simulink model "model_sim_CHB5_36_new_temp"  (R2020a)
settings: Solver=FixedStepAuto  StartTime=0.0  StopTime=5  RelTol=1e-3
InitFcn:
  | sysinit
values from neighbouring files (symbols this model uses):
  C = 0.03    [sysinit.m]
  C_f = 0.625e-6    (= 6.25e-07)    [sysinit.m]
  f = 50    [sysinit.m]
  f_switch = 500    [sysinit.m]
  L = 0.004    [sysinit.m]
  L_f = 3e-6    (= 3e-06)    [sysinit.m]
  R = 1.2    [sysinit.m]
  R_f = 1.5    [sysinit.m]
  Rth_h = 7.5e-3    (= 0.0075)    [Device_Parameter.m]
  Rth_h_tau = 0.5    [Device_Parameter.m]
  st = 5e-7    (= 5e-07)    [sysinit.m]
  temp_init = 40    [sysinit.m]
  Ts = 1e-6    (= 1e-06)    [sysinit.m]
  Ts2 = 0.5E-3    (= 0.0005)    [sysinit.m]
  Udc = 2500    [sysinit.m]
undefined symbols (not defined in the file or in its folder): DIODE_204520, DIODE_344520, DIODE_D1031SH, DIODE_D1331SH, IGCT_364520_36, IGCT_364521_36, IGCT_654522_6, magnitude, Ts1
libraries: powerlib x278, powerlib_meascontrol x84, simulink x9
(part 2 of 5)

== system model_sim_CHB5_36_new_temp/MAIN TOPOLOGY level-5/IGCT4 ==
  PWM : Inport
  Current Measurement1 : powerlib/Measurements/Current Measurement  PhasorSimulation=off  OutputType=Complex  PSBequivalent=0
  Demux : Demux
  Diode{1..3,6,8} (5 alike) : powerlib/Power Electronics/Diode  Ron=rto  Lon=0  Vf=vto  IC=0  UseSnubber=off  Rs=500  Cs=250e-9  Measurements=on
  IGBT{,1..3} (4 alike) : powerlib/Power Electronics/IGBT  Ron=rt  Lon=0  Vf=vt  Tf=1e-6  Tt=2e-6  IC=0  Rs=1e5  Cs=inf  Measurements=on
  Series RLC Branch1 : powerlib/Elements/Series RLC Branch  LConnTagsString=__new0  RConnTagsString=__new0  BranchType=RL  Resistance=1e-5  Inductance=3.0E-6  SetiL0=off  InitialCurrent=0  Capacitance=1e-6  Setx0=off  InitialVoltage=0  Measurements=None
  Series RLC Branch10 : powerlib/Elements/Series RLC Branch  LConnTagsString=__new0  RConnTagsString=__new0  BranchType=L  Resistance=1  Inductance=0.4e-6  SetiL0=off  InitialCurrent=0  Capacitance=1e-6  Setx0=off  InitialVoltage=0  Measurements=None
  Series RLC Branch12 : powerlib/Elements/Series RLC Branch  LConnTagsString=__new0  RConnTagsString=__new0  BranchType=RL  Resistance=1e-5  Inductance=1E-9  SetiL0=off  InitialCurrent=0  Capacitance=1e-6  Setx0=off  InitialVoltage=0  Measurements=None
  Series RLC Branch14 : powerlib/Elements/Series RLC Branch  LConnTagsString=__new0  RConnTagsString=__new0  BranchType=L  Resistance=1  Inductance=1E-7  SetiL0=off  InitialCurrent=0  Capacitance=1e-6  Setx0=off  InitialVoltage=0  Measurements=None
  Series RLC Branch2 : powerlib/Elements/Series RLC Branch  LConnTagsString=__new0  RConnTagsString=__new0  BranchType=RC  Resistance=1e-5  Inductance=20e-6  SetiL0=off  InitialCurrent=0  Capacitance=17e-6  Setx0=off  InitialVoltage=0  Measurements=None
  Series RLC Branch3 : powerlib/Elements/Series RLC Branch  LConnTagsString=__new0  RConnTagsString=__new0  BranchType=RL  Resistance=1e-5  Inductance=1E-9  SetiL0=off  InitialCurrent=0  Capacitance=1e-6  Setx0=off  InitialVoltage=0  Measurements=None
  Series RLC Branch5 : powerlib/Elements/Series RLC Branch  LConnTagsString=__new0  RConnTagsString=__new0  BranchType=L  Resistance=1  Inductance=1E-7  SetiL0=off  InitialCurrent=0  Capacitance=1e-6  Setx0=off  InitialVoltage=0  Measurements=None
  Series RLC Branch7 : powerlib/Elements/Series RLC Branch  LConnTagsString=__new0  RConnTagsString=__new0  BranchType=RL  Resistance=0.6  Inductance=1e-6  SetiL0=off  InitialCurrent=0  Capacitance=1e-6  Setx0=off  InitialVoltage=0  Measurements=None
  Series RLC Branch9 : powerlib/Elements/Series RLC Branch  LConnTagsString=__new0  RConnTagsString=__new0  BranchType=L  Resistance=1  Inductance=0.4e-6  SetiL0=off  InitialCurrent=0  Capacitance=1e-6  Setx0=off  InitialVoltage=0  Measurements=None
  Terminator{,1..9} (10 alike) : Terminator
  Udc+ : PMIOPort  Side=Left
  udc- : PMIOPort  Port=2  Side=Left
  p1 : PMIOPort  Port=3  Side=Right
  p2 : PMIOPort  Port=4  Side=Right
  wires:
  Diode3/1 -> Terminator9/1
  IGBT3/1 -> Terminator5/1
  [n1] -> IGBT3/1
  IGBT1/1 -> Terminator4/1
  IGBT2/1 -> Terminator3/1
  IGBT/1 -> Terminator2/1
  [n2] -> IGBT1/1
  [p1] -> IGBT2/1
  Current Measurement1/1 -> Terminator/1
  Diode2/1 -> Terminator8/1
  [p2] -> IGBT/1
  Diode8/1 -> Terminator7/1
  Diode1/1 -> Terminator6/1
  Diode6/1 -> Terminator1/1
  Demux/3 -> [n2]
  PWM/1 -> Demux/1
  Demux/1 -> [p2]
  Demux/2 -> [p1]
  Demux/4 -> [n1]
  connections:
  Series RLC Branch10/LConn1 -- udc-/RConn1
  Series RLC Branch9/LConn1 -- Udc+/RConn1
  Diode6/RConn1 -- Series RLC Branch7/RConn1 -- Series RLC Branch2/LConn1
  Current Measurement1/LConn1 -- Series RLC Branch1/RConn1 -- Series RLC Branch3/LConn1 -- Series RLC Branch12/LConn1
  Diode3/LConn1 -- IGBT3/RConn1 -- Series RLC Branch14/RConn1
  Series RLC Branch3/RConn1 -- IGBT/LConn1 -- Diode8/RConn1
  Diode1/LConn1 -- Series RLC Branch5/RConn1 -- IGBT1/RConn1
  Current Measurement1/RConn1 -- Diode6/LConn1
  Diode2/RConn1 -- Series RLC Branch12/RConn1 -- IGBT2/LConn1
  p1/RConn1 -- Diode2/LConn1 -- Diode3/RConn1 -- IGBT3/LConn1 -- IGBT2/RConn1
  Series RLC Branch5/LConn1 -- Series RLC Branch14/LConn1 -- Series RLC Branch10/RConn1 -- Series RLC Branch2/RConn1
  Series RLC Branch1/LConn1 -- Series RLC Branch7/LConn1 -- Series RLC Branch9/RConn1
  p2/RConn1 -- IGBT1/LConn1 -- Diode1/RConn1 -- Diode8/LConn1 -- IGBT/RConn1

== system model_sim_CHB5_36_new_temp/MAIN TOPOLOGY level-5/IGCT5 ==
  PWM : Inport
  Current Measurement1 : powerlib/Measurements/Current Measurement  PhasorSimulation=off  OutputType=Complex  PSBequivalent=0
  Demux : Demux
  Diode{1..3,6,8} (5 alike) : powerlib/Power Electronics/Diode  Ron=rto  Lon=0  Vf=vto  IC=0  UseSnubber=off  Rs=500  Cs=250e-9  Measurements=on
  IGBT{,1..3} (4 alike) : powerlib/Power Electronics/IGBT  Ron=rt  Lon=0  Vf=vt  Tf=1e-6  Tt=2e-6  IC=0  Rs=1e5  Cs=inf  Measurements=on
  Series RLC Branch1 : powerlib/Elements/Series RLC Branch  LConnTagsString=__new0  RConnTagsString=__new0  BranchType=RL  Resistance=1e-5  Inductance=3.0E-6  SetiL0=off  InitialCurrent=0  Capacitance=1e-6  Setx0=off  InitialVoltage=0  Measurements=None
  Series RLC Branch10 : powerlib/Elements/Series RLC Branch  LConnTagsString=__new0  RConnTagsString=__new0  BranchType=L  Resistance=1  Inductance=0.4e-6  SetiL0=off  InitialCurrent=0  Capacitance=1e-6  Setx0=off  InitialVoltage=0  Measurements=None
  Series RLC Branch12 : powerlib/Elements/Series RLC Branch  LConnTagsString=__new0  RConnTagsString=__new0  BranchType=RL  Resistance=1e-5  Inductance=1E-9  SetiL0=off  InitialCurrent=0  Capacitance=1e-6  Setx0=off  InitialVoltage=0  Measurements=None
  Series RLC Branch14 : powerlib/Elements/Series RLC Branch  LConnTagsString=__new0  RConnTagsString=__new0  BranchType=L  Resistance=1  Inductance=1E-7  SetiL0=off  InitialCurrent=0  Capacitance=1e-6  Setx0=off  InitialVoltage=0  Measurements=None
  Series RLC Branch2 : powerlib/Elements/Series RLC Branch  LConnTagsString=__new0  RConnTagsString=__new0  BranchType=RC  Resistance=1e-5  Inductance=20e-6  SetiL0=off  InitialCurrent=0  Capacitance=17e-6  Setx0=off  InitialVoltage=0  Measurements=None
  Series RLC Branch3 : powerlib/Elements/Series RLC Branch  LConnTagsString=__new0  RConnTagsString=__new0  BranchType=RL  Resistance=1e-5  Inductance=1E-9  SetiL0=off  InitialCurrent=0  Capacitance=1e-6  Setx0=off  InitialVoltage=0  Measurements=None
  Series RLC Branch5 : powerlib/Elements/Series RLC Branch  LConnTagsString=__new0  RConnTagsString=__new0  BranchType=L  Resistance=1  Inductance=1E-7  SetiL0=off  InitialCurrent=0  Capacitance=1e-6  Setx0=off  InitialVoltage=0  Measurements=None
  Series RLC Branch7 : powerlib/Elements/Series RLC Branch  LConnTagsString=__new0  RConnTagsString=__new0  BranchType=RL  Resistance=0.6  Inductance=1e-6  SetiL0=off  InitialCurrent=0  Capacitance=1e-6  Setx0=off  InitialVoltage=0  Measurements=None
  Series RLC Branch9 : powerlib/Elements/Series RLC Branch  LConnTagsString=__new0  RConnTagsString=__new0  BranchType=L  Resistance=1  Inductance=0.4e-6  SetiL0=off  InitialCurrent=0  Capacitance=1e-6  Setx0=off  InitialVoltage=0  Measurements=None
  Terminator{,1..9} (10 alike) : Terminator
  Udc+ : PMIOPort  Side=Left
  udc- : PMIOPort  Port=2  Side=Left
  p1 : PMIOPort  Port=3  Side=Right
  p2 : PMIOPort  Port=4  Side=Right
  wires:
  Diode3/1 -> Terminator9/1
  IGBT3/1 -> Terminator5/1
  [n1] -> IGBT3/1
  IGBT1/1 -> Terminator4/1
  IGBT2/1 -> Terminator3/1
  IGBT/1 -> Terminator2/1
  [n2] -> IGBT1/1
  [p1] -> IGBT2/1
  Current Measurement1/1 -> Terminator/1
  Diode2/1 -> Terminator8/1
  [p2] -> IGBT/1
  Diode8/1 -> Terminator7/1
  Diode1/1 -> Terminator6/1
  Diode6/1 -> Terminator1/1
  Demux/3 -> [n2]
  PWM/1 -> Demux/1
  Demux/1 -> [p2]
  Demux/2 -> [p1]
  Demux/4 -> [n1]
  connections:
  Series RLC Branch10/LConn1 -- udc-/RConn1
  Series RLC Branch9/LConn1 -- Udc+/RConn1
  Diode6/RConn1 -- Series RLC Branch7/RConn1 -- Series RLC Branch2/LConn1
  Current Measurement1/LConn1 -- Series RLC Branch1/RConn1 -- Series RLC Branch3/LConn1 -- Series RLC Branch12/LConn1
  Diode3/LConn1 -- IGBT3/RConn1 -- Series RLC Branch14/RConn1
  Series RLC Branch3/RConn1 -- IGBT/LConn1 -- Diode8/RConn1
  Diode1/LConn1 -- Series RLC Branch5/RConn1 -- IGBT1/RConn1
  Current Measurement1/RConn1 -- Diode6/LConn1
  Diode2/RConn1 -- Series RLC Branch12/RConn1 -- IGBT2/LConn1
  p1/RConn1 -- Diode2/LConn1 -- Diode3/RConn1 -- IGBT3/LConn1 -- IGBT2/RConn1
  Series RLC Branch5/LConn1 -- Series RLC Branch14/LConn1 -- Series RLC Branch10/RConn1 -- Series RLC Branch2/RConn1
  Series RLC Branch1/LConn1 -- Series RLC Branch7/LConn1 -- Series RLC Branch9/RConn1
  p2/RConn1 -- IGBT1/LConn1 -- Diode1/RConn1 -- Diode8/LConn1 -- IGBT/RConn1

== system model_sim_CHB5_36_new_temp/MAIN TOPOLOGY level-5/IGCT6 ==
  PWM : Inport
  Current Measurement1 : powerlib/Measurements/Current Measurement  PhasorSimulation=off  OutputType=Complex  PSBequivalent=0
  Demux : Demux
  Diode{1..3,6,8} (5 alike) : powerlib/Power Electronics/Diode  Ron=rto  Lon=0  Vf=vto  IC=0  UseSnubber=off  Rs=500  Cs=250e-9  Measurements=on
  IGBT{,1..3} (4 alike) : powerlib/Power Electronics/IGBT  Ron=rt  Lon=0  Vf=vt  Tf=1e-6  Tt=2e-6  IC=0  Rs=1e5  Cs=inf  Measurements=on
  Series RLC Branch1 : powerlib/Elements/Series RLC Branch  LConnTagsString=__new0  RConnTagsString=__new0  BranchType=RL  Resistance=1e-5  Inductance=3.0E-6  SetiL0=off  InitialCurrent=0  Capacitance=1e-6  Setx0=off  InitialVoltage=0  Measurements=None
  Series RLC Branch10 : powerlib/Elements/Series RLC Branch  LConnTagsString=__new0  RConnTagsString=__new0  BranchType=L  Resistance=1  Inductance=0.4e-6  SetiL0=off  InitialCurrent=0  Capacitance=1e-6  Setx0=off  InitialVoltage=0  Measurements=None
  Series RLC Branch12 : powerlib/Elements/Series RLC Branch  LConnTagsString=__new0  RConnTagsString=__new0  BranchType=RL  Resistance=1e-5  Inductance=1E-9  SetiL0=off  InitialCurrent=0  Capacitance=1e-6  Setx0=off  InitialVoltage=0  Measurements=None
  Series RLC Branch14 : powerlib/Elements/Series RLC Branch  LConnTagsString=__new0  RConnTagsString=__new0  BranchType=L  Resistance=1  Inductance=1E-7  SetiL0=off  InitialCurrent=0  Capacitance=1e-6  Setx0=off  InitialVoltage=0  Measurements=None
  Series RLC Branch2 : powerlib/Elements/Series RLC Branch  LConnTagsString=__new0  RConnTagsString=__new0  BranchType=RC  Resistance=1e-5  Inductance=20e-6  SetiL0=off  InitialCurrent=0  Capacitance=17e-6  Setx0=off  InitialVoltage=0  Measurements=None
  Series RLC Branch3 : powerlib/Elements/Series RLC Branch  LConnTagsString=__new0  RConnTagsString=__new0  BranchType=RL  Resistance=1e-5  Inductance=1E-9  SetiL0=off  InitialCurrent=0  Capacitance=1e-6  Setx0=off  InitialVoltage=0  Measurements=None
  Series RLC Branch5 : powerlib/Elements/Series RLC Branch  LConnTagsString=__new0  RConnTagsString=__new0  BranchType=L  Resistance=1  Inductance=1E-7  SetiL0=off  InitialCurrent=0  Capacitance=1e-6  Setx0=off  InitialVoltage=0  Measurements=None
  Series RLC Branch7 : powerlib/Elements/Series RLC Branch  LConnTagsString=__new0  RConnTagsString=__new0  BranchType=RL  Resistance=0.6  Inductance=1e-6  SetiL0=off  InitialCurrent=0  Capacitance=1e-6  Setx0=off  InitialVoltage=0  Measurements=None
  Series RLC Branch9 : powerlib/Elements/Series RLC Branch  LConnTagsString=__new0  RConnTagsString=__new0  BranchType=L  Resistance=1  Inductance=0.4e-6  SetiL0=off  InitialCurrent=0  Capacitance=1e-6  Setx0=off  InitialVoltage=0  Measurements=None
  Terminator{,1..9} (10 alike) : Terminator
  Udc+ : PMIOPort  Side=Left
  udc- : PMIOPort  Port=2  Side=Left
  p1 : PMIOPort  Port=3  Side=Right
  p2 : PMIOPort  Port=4  Side=Right
  wires:
  Demux/4 -> [n1]
  Demux/2 -> [p1]
  Demux/1 -> [p2]
  PWM/1 -> Demux/1
  Demux/3 -> [n2]
  Diode6/1 -> Terminator1/1
  Diode1/1 -> Terminator6/1
  Diode8/1 -> Terminator7/1
  [p2] -> IGBT/1
  Diode2/1 -> Terminator8/1
  Current Measurement1/1 -> Terminator/1
  [p1] -> IGBT2/1
  [n2] -> IGBT1/1
  IGBT/1 -> Terminator2/1
  IGBT2/1 -> Terminator3/1
  IGBT1/1 -> Terminator4/1
  [n1] -> IGBT3/1
  IGBT3/1 -> Terminator5/1
  Diode3/1 -> Terminator9/1
  connections:
  IGBT/RConn1 -- Diode8/LConn1 -- Diode1/RConn1 -- IGBT1/LConn1 -- p2/RConn1
  Series RLC Branch9/RConn1 -- Series RLC Branch7/LConn1 -- Series RLC Branch1/LConn1
  Series RLC Branch2/RConn1 -- Series RLC Branch10/RConn1 -- Series RLC Branch14/LConn1 -- Series RLC Branch5/LConn1
  IGBT2/RConn1 -- IGBT3/LConn1 -- Diode3/RConn1 -- Diode2/LConn1 -- p1/RConn1
  IGBT2/LConn1 -- Series RLC Branch12/RConn1 -- Diode2/RConn1
  Current Measurement1/RConn1 -- Diode6/LConn1
  IGBT1/RConn1 -- Series RLC Branch5/RConn1 -- Diode1/LConn1
  Diode8/RConn1 -- IGBT/LConn1 -- Series RLC Branch3/RConn1
  Series RLC Branch14/RConn1 -- IGBT3/RConn1 -- Diode3/LConn1
  Series RLC Branch12/LConn1 -- Series RLC Branch3/LConn1 -- Series RLC Branch1/RConn1 -- Current Measurement1/LConn1
  Series RLC Branch2/LConn1 -- Series RLC Branch7/RConn1 -- Diode6/RConn1
  Series RLC Branch9/LConn1 -- Udc+/RConn1
  Series RLC Branch10/LConn1 -- udc-/RConn1

== system model_sim_CHB5_36_new_temp/MAIN TOPOLOGY level-5/Subsystem2 ==
  Zigzag Phase-Shifting Transformer : powerlib/Elements/Zigzag Phase-Shifting Transformer  SecondaryConnection=Delta D1(-30 deg.)  SetSaturation=off  SetInitialFlux=off  Measurements=None  UNITS=pu  NominalPower=[ p 50]  PrimaryVoltage=vp  SecondaryVoltage="[ vs  +5]"  Winding1=windingpri  Winding2=windingpri  Winding3=windingsec  RmLm=mag  Rm=500  Saturation=[ 0,0 ; 0.0024,1.2 ; 1.0,1.52 ]  InitialFluxes=[0,0,0]  BreakLoop=off  DiscreteSolver=Trapezoidal iterative  DataType=off
  Zigzag Phase-Shifting Transformer1 : powerlib/Elements/Zigzag Phase-Shifting Transformer  SecondaryConnection=Delta D1(-30 deg.)  SetSaturation=off  SetInitialFlux=off  Measurements=None  UNITS=pu  NominalPower=[ p 50]  PrimaryVoltage=vp  SecondaryVoltage="[ vs  +15]"  Winding1=windingpri  Winding2=windingpri  Winding3=windingsec  RmLm=mag  Rm=500  Saturation=[ 0,0 ; 0.0024,1.2 ; 1.0,1.52 ]  InitialFluxes=[0,0,0]  BreakLoop=off  DiscreteSolver=Trapezoidal iterative  DataType=off
  Zigzag Phase-Shifting Transformer2 : powerlib/Elements/Zigzag Phase-Shifting Transformer  SecondaryConnection=Delta D1(-30 deg.)  SetSaturation=off  SetInitialFlux=off  Measurements=None  UNITS=pu  NominalPower=[ p 50]  PrimaryVoltage=vp  SecondaryVoltage="[ vs  +25]"  Winding1=windingpri  Winding2=windingpri  Winding3=windingsec  RmLm=mag  Rm=500  Saturation=[ 0,0 ; 0.0024,1.2 ; 1.0,1.52 ]  InitialFluxes=[0,0,0]  BreakLoop=off  DiscreteSolver=Trapezoidal iterative  DataType=off
  Zigzag Phase-Shifting Transformer3 : powerlib/Elements/Zigzag Phase-Shifting Transformer  SecondaryConnection=Delta D1(-30 deg.)  SetSaturation=off  SetInitialFlux=off  Measurements=None  UNITS=pu  NominalPower=[ p 50]  PrimaryVoltage=vp  SecondaryVoltage="[ vs  -25]"  Winding1=windingpri  Winding2=windingpri  Winding3=windingsec  RmLm=mag  Rm=500  Saturation=[ 0,0 ; 0.0024,1.2 ; 1.0,1.52 ]  InitialFluxes=[0,0,0]  BreakLoop=off  DiscreteSolver=Trapezoidal iterative  DataType=off
  Zigzag Phase-Shifting Transformer4 : powerlib/Elements/Zigzag Phase-Shifting Transformer  SecondaryConnection=Delta D1(-30 deg.)  SetSaturation=off  SetInitialFlux=off  Measurements=None  UNITS=pu  NominalPower=[ p 50]  PrimaryVoltage=vp  SecondaryVoltage="[ vs  -5]"  Winding1=windingpri  Winding2=windingpri  Winding3=windingsec  RmLm=mag  Rm=500  Saturation=[ 0,0 ; 0.0024,1.2 ; 1.0,1.52 ]  InitialFluxes=[0,0,0]  BreakLoop=off  DiscreteSolver=Trapezoidal iterative  DataType=off
  Zigzag Phase-Shifting Transformer5 : powerlib/Elements/Zigzag Phase-Shifting Transformer  SecondaryConnection=Delta D1(-30 deg.)  SetSaturation=off  SetInitialFlux=off  Measurements=None  UNITS=pu  NominalPower=[ p 50]  PrimaryVoltage=vp  SecondaryVoltage="[ vs  -15]"  Winding1=windingpri  Winding2=windingpri  Winding3=windingsec  RmLm=mag  Rm=500  Saturation=[ 0,0 ; 0.0024,1.2 ; 1.0,1.52 ]  InitialFluxes=[0,0,0]  BreakLoop=off  DiscreteSolver=Trapezoidal iterative  DataType=off
  output Ground1 : powerlib/Elements/Ground  LConnTagsString=a  RConnTagsString=__newr0
  A : PMIOPort  Side=Left
  a+5 : PMIOPort  Port=2  Side=Right
  B : PMIOPort  Port=3  Side=Left
  C : PMIOPort  Port=4  Side=Left
  b+5 : PMIOPort  Port=5  Side=Right
  c+5 : PMIOPort  Port=6  Side=Right
  a-25 : PMIOPort  Port=7  Side=Right
  b-25 : PMIOPort  Port=8  Side=Right
  c-25 : PMIOPort  Port=9  Side=Right
  a+15 : PMIOPort  Port=10  Side=Right
  b+15 : PMIOPort  Port=11  Side=Right
  c+15 : PMIOPort  Port=12  Side=Right
  a-15 : PMIOPort  Port=13  Side=Right
  b-15 : PMIOPort  Port=14  Side=Right
  c-15 : PMIOPort  Port=15  Side=Right
  a25 : PMIOPort  Port=16  Side=Right
  b25 : PMIOPort  Port=17  Side=Right
  c25 : PMIOPort  Port=18  Side=Right
  a-5 : PMIOPort  Port=19  Side=Right
  b-5 : PMIOPort  Port=20  Side=Right
  c-5 : PMIOPort  Port=21  Side=Right
  connections:
  Zigzag Phase-Shifting Transformer4/LConn4 -- Zigzag Phase-Shifting Transformer4/LConn5 -- output Ground1/LConn1 -- Zigzag Phase-Shifting Transformer4/LConn6
  b+5/RConn1 -- Zigzag Phase-Shifting Transformer/RConn2
  a+5/RConn1 -- Zigzag Phase-Shifting Transformer/RConn1
  c+5/RConn1 -- Zigzag Phase-Shifting Transformer/RConn3
  c-25/RConn1 -- Zigzag Phase-Shifting Transformer3/RConn3
  b-25/RConn1 -- Zigzag Phase-Shifting Transformer3/RConn2
  a-25/RConn1 -- Zigzag Phase-Shifting Transformer3/RConn1
  c+15/RConn1 -- Zigzag Phase-Shifting Transformer1/RConn3
  b+15/RConn1 -- Zigzag Phase-Shifting Transformer1/RConn2
  a+15/RConn1 -- Zigzag Phase-Shifting Transformer1/RConn1
  c-15/RConn1 -- Zigzag Phase-Shifting Transformer5/RConn3
  b-15/RConn1 -- Zigzag Phase-Shifting Transformer5/RConn2
  a-15/RConn1 -- Zigzag Phase-Shifting Transformer5/RConn1
  c25/RConn1 -- Zigzag Phase-Shifting Transformer2/RConn3
  b25/RConn1 -- Zigzag Phase-Shifting Transformer2/RConn2
  a25/RConn1 -- Zigzag Phase-Shifting Transformer2/RConn1
  c-5/RConn1 -- Zigzag Phase-Shifting Transformer4/RConn3
  b-5/RConn1 -- Zigzag Phase-Shifting Transformer4/RConn2
  a-5/RConn1 -- Zigzag Phase-Shifting Transformer4/RConn1
  Zigzag Phase-Shifting Transformer2/LConn6 -- Zigzag Phase-Shifting Transformer4/LConn3
  Zigzag Phase-Shifting Transformer3/LConn6 -- Zigzag Phase-Shifting Transformer1/LConn3
  Zigzag Phase-Shifting Transformer1/LConn6 -- Zigzag Phase-Shifting Transformer5/LConn3
  Zigzag Phase-Shifting Transformer5/LConn6 -- Zigzag Phase-Shifting Transformer2/LConn3
  Zigzag Phase-Shifting Transformer/LConn2 -- B/RConn1
  Zigzag Phase-Shifting Transformer/LConn4 -- Zigzag Phase-Shifting Transformer3/LConn1
  Zigzag Phase-Shifting Transformer/LConn5 -- Zigzag Phase-Shifting Transformer3/LConn2
  Zigzag Phase-Shifting Transformer/LConn6 -- Zigzag Phase-Shifting Transformer3/LConn3
  Zigzag Phase-Shifting Transformer3/LConn4 -- Zigzag Phase-Shifting Transformer1/LConn1
  Zigzag Phase-Shifting Transformer3/LConn5 -- Zigzag Phase-Shifting Transformer1/LConn2
  Zigzag Phase-Shifting Transformer1/LConn4 -- Zigzag Phase-Shifting Transformer5/LConn1
  Zigzag Phase-Shifting Transformer1/LConn5 -- Zigzag Phase-Shifting Transformer5/LConn2
  Zigzag Phase-Shifting Transformer5/LConn4 -- Zigzag Phase-Shifting Transformer2/LConn1
  Zigzag Phase-Shifting Transformer5/LConn5 -- Zigzag Phase-Shifting Transformer2/LConn2
  Zigzag Phase-Shifting Transformer2/LConn4 -- Zigzag Phase-Shifting Transformer4/LConn1
  Zigzag Phase-Shifting Transformer4/LConn2 -- Zigzag Phase-Shifting Transformer2/LConn5
  C/RConn1 -- Zigzag Phase-Shifting Transformer/LConn3
  A/RConn1 -- Zigzag Phase-Shifting Transformer/LConn1

== system model_sim_CHB5_36_new_temp/MAIN TOPOLOGY level-5/VOLTAGE_MEASURE ==
  Voltage Measurement{1..6} (6 alike) : powerlib/Measurements/Voltage Measurement  PhasorSimulation=off  OutputType=Complex  PSBequivalent=0
  N : PMIOPort  Side=Left
  A : PMIOPort  Port=2  Side=Left
  B : PMIOPort  Port=3  Side=Right
  C : PMIOPort  Port=4  Side=Right
  tag scope: VloadABline=global, VloadAphase=global, VloadBCline=global, VloadBphase=global, VloadCAline=global, VloadCphase=global
  wires:
  Voltage Measurement2/1 -> [VloadAphase]
  Voltage Measurement4/1 -> [VloadBphase]
  Voltage Measurement5/1 -> [VloadCAline]
  Voltage Measurement3/1 -> [VloadBCline]
  Voltage Measurement1/1 -> [VloadABline]
  Voltage Measurement6/1 -> [VloadCphase]
  connections:
  Voltage Measurement2/LConn2 -- Voltage Measurement6/LConn2 -- Voltage Measurement4/LConn2 -- N/RConn1
  Voltage Measurement6/LConn1 -- Voltage Measurement5/LConn1 -- Voltage Measurement3/LConn2 -- C/RConn1
  Voltage Measurement3/LConn1 -- Voltage Measurement1/LConn2 -- B/RConn1 -- Voltage Measurement4/LConn1
  Voltage Measurement5/LConn2 -- Voltage Measurement1/LConn1 -- Voltage Measurement2/LConn1 -- A/RConn1

== system model_sim_CHB5_36_new_temp/Subsystem/IGCT1 ==
  PWM : Inport
  Current Measurement1 : powerlib/Measurements/Current Measurement  PhasorSimulation=off  OutputType=Complex  PSBequivalent=0
  Demux : Demux
  Diode{1..3,6,8} (5 alike) : powerlib/Power Electronics/Diode  Ron=DIODE.rF  Lon=0  Vf=DIODE.VF0  IC=0  UseSnubber=off  Rs=500  Cs=250e-9  Measurements=on
  IGBT{,1..3} (4 alike) : powerlib/Power Electronics/IGBT  Ron=IGCT.rT  Lon=0  Vf=IGCT.VT0  Tf=1e-6  Tt=2e-6  IC=0  Rs=1e5  Cs=inf  Measurements=on
  Series RLC Branch1 : powerlib/Elements/Series RLC Branch  LConnTagsString=__new0  RConnTagsString=__new0  BranchType=RL  Resistance=1e-5  Inductance=3.0E-6  SetiL0=off  InitialCurrent=0  Capacitance=1e-6  Setx0=off  InitialVoltage=0  Measurements=None
  Series RLC Branch10 : powerlib/Elements/Series RLC Branch  LConnTagsString=__new0  RConnTagsString=__new0  BranchType=L  Resistance=1  Inductance=0.4e-6  SetiL0=off  InitialCurrent=0  Capacitance=1e-6  Setx0=off  InitialVoltage=0  Measurements=None
  Series RLC Branch12 : powerlib/Elements/Series RLC Branch  LConnTagsString=__new0  RConnTagsString=__new0  BranchType=RL  Resistance=1e-5  Inductance=1E-9  SetiL0=off  InitialCurrent=0  Capacitance=1e-6  Setx0=off  InitialVoltage=0  Measurements=None
  Series RLC Branch14 : powerlib/Elements/Series RLC Branch  LConnTagsString=__new0  RConnTagsString=__new0  BranchType=L  Resistance=1  Inductance=1E-7  SetiL0=off  InitialCurrent=0  Capacitance=1e-6  Setx0=off  InitialVoltage=0  Measurements=None
  Series RLC Branch2 : powerlib/Elements/Series RLC Branch  LConnTagsString=__new0  RConnTagsString=__new0  BranchType=RC  Resistance=1e-5  Inductance=20e-6  SetiL0=off  InitialCurrent=0  Capacitance=17e-6  Setx0=off  InitialVoltage=0  Measurements=None
  Series RLC Branch3 : powerlib/Elements/Series RLC Branch  LConnTagsString=__new0  RConnTagsString=__new0  BranchType=RL  Resistance=1e-5  Inductance=1E-9  SetiL0=off  InitialCurrent=0  Capacitance=1e-6  Setx0=off  InitialVoltage=0  Measurements=None
  Series RLC Branch5 : powerlib/Elements/Series RLC Branch  LConnTagsString=__new0  RConnTagsString=__new0  BranchType=L  Resistance=1  Inductance=1E-7  SetiL0=off  InitialCurrent=0  Capacitance=1e-6  Setx0=off  InitialVoltage=0  Measurements=None
  Series RLC Branch7 : powerlib/Elements/Series RLC Branch  LConnTagsString=__new0  RConnTagsString=__new0  BranchType=RL  Resistance=0.6  Inductance=1e-6  SetiL0=off  InitialCurrent=0  Capacitance=1e-6  Setx0=off  InitialVoltage=0  Measurements=None
  Series RLC Branch9 : powerlib/Elements/Series RLC Branch  LConnTagsString=__new0  RConnTagsString=__new0  BranchType=L  Resistance=1  Inductance=0.4e-6  SetiL0=off  InitialCurrent=0  Capacitance=1e-6  Setx0=off  InitialVoltage=0  Measurements=None
  Terminator{,1..9} (10 alike) : Terminator
  Udc+ : PMIOPort  Side=Left
  udc- : PMIOPort  Port=2  Side=Left
  p1 : PMIOPort  Port=3  Side=Right
  p2 : PMIOPort  Port=4  Side=Right
  wires:
  Diode3/1 -> Terminator9/1
  IGBT3/1 -> Terminator5/1
  [n1] -> IGBT3/1
  IGBT1/1 -> Terminator4/1
  IGBT2/1 -> Terminator3/1
  IGBT/1 -> Terminator2/1
  [n2] -> IGBT1/1
  [p1] -> IGBT2/1
  Current Measurement1/1 -> Terminator/1
  Diode2/1 -> Terminator8/1
  [p2] -> IGBT/1
  Diode8/1 -> Terminator7/1
  Diode1/1 -> Terminator6/1
  Diode6/1 -> Terminator1/1
  Demux/3 -> [n2]
  PWM/1 -> Demux/1
  Demux/1 -> [p2]
  Demux/2 -> [p1]
  Demux/4 -> [n1]
  connections:
  Series RLC Branch10/LConn1 -- udc-/RConn1
  Series RLC Branch9/LConn1 -- Udc+/RConn1
  Diode6/RConn1 -- Series RLC Branch7/RConn1 -- Series RLC Branch2/LConn1
  Current Measurement1/LConn1 -- Series RLC Branch1/RConn1 -- Series RLC Branch3/LConn1 -- Series RLC Branch12/LConn1
  Series RLC Branch14/RConn1 -- Diode3/LConn1 -- IGBT3/RConn1
  Series RLC Branch3/RConn1 -- IGBT/LConn1 -- Diode8/RConn1
  Series RLC Branch5/RConn1 -- Diode1/LConn1 -- IGBT1/RConn1
  Current Measurement1/RConn1 -- Diode6/LConn1
  Series RLC Branch12/RConn1 -- IGBT2/LConn1 -- Diode2/RConn1
  p1/RConn1 -- Diode3/RConn1 -- IGBT3/LConn1 -- IGBT2/RConn1 -- Diode2/LConn1
  Series RLC Branch5/LConn1 -- Series RLC Branch14/LConn1 -- Series RLC Branch10/RConn1 -- Series RLC Branch2/RConn1
  Series RLC Branch1/LConn1 -- Series RLC Branch7/LConn1 -- Series RLC Branch9/RConn1
  p2/RConn1 -- Diode1/RConn1 -- IGBT1/LConn1 -- Diode8/LConn1 -- IGBT/RConn1

== system model_sim_CHB5_36_new_temp/Subsystem/IGCT2 ==
  PWM : Inport
  Current Measurement1 : powerlib/Measurements/Current Measurement  PhasorSimulation=off  OutputType=Complex  PSBequivalent=0
  Demux : Demux
  Diode{1..3,6,8} (5 alike) : powerlib/Power Electronics/Diode  Ron=DIODE.rF  Lon=0  Vf=DIODE.VF0  IC=0  UseSnubber=off  Rs=500  Cs=250e-9  Measurements=on
  IGBT{,1..3} (4 alike) : powerlib/Power Electronics/IGBT  Ron=IGCT.rT  Lon=0  Vf=IGCT.VT0  Tf=1e-6  Tt=2e-6  IC=0  Rs=1e5  Cs=inf  Measurements=on
  Series RLC Branch1 : powerlib/Elements/Series RLC Branch  LConnTagsString=__new0  RConnTagsString=__new0  BranchType=RL  Resistance=1e-5  Inductance=3.0E-6  SetiL0=off  InitialCurrent=0  Capacitance=1e-6  Setx0=off  InitialVoltage=0  Measurements=None
  Series RLC Branch10 : powerlib/Elements/Series RLC Branch  LConnTagsString=__new0  RConnTagsString=__new0  BranchType=L  Resistance=1  Inductance=0.4e-6  SetiL0=off  InitialCurrent=0  Capacitance=1e-6  Setx0=off  InitialVoltage=0  Measurements=None
  Series RLC Branch12 : powerlib/Elements/Series RLC Branch  LConnTagsString=__new0  RConnTagsString=__new0  BranchType=RL  Resistance=1e-5  Inductance=1E-9  SetiL0=off  InitialCurrent=0  Capacitance=1e-6  Setx0=off  InitialVoltage=0  Measurements=None
  Series RLC Branch14 : powerlib/Elements/Series RLC Branch  LConnTagsString=__new0  RConnTagsString=__new0  BranchType=L  Resistance=1  Inductance=1E-7  SetiL0=off  InitialCurrent=0  Capacitance=1e-6  Setx0=off  InitialVoltage=0  Measurements=None
  Series RLC Branch2 : powerlib/Elements/Series RLC Branch  LConnTagsString=__new0  RConnTagsString=__new0  BranchType=RC  Resistance=1e-5  Inductance=20e-6  SetiL0=off  InitialCurrent=0  Capacitance=17e-6  Setx0=off  InitialVoltage=0  Measurements=None
  Series RLC Branch3 : powerlib/Elements/Series RLC Branch  LConnTagsString=__new0  RConnTagsString=__new0  BranchType=RL  Resistance=1e-5  Inductance=1E-9  SetiL0=off  InitialCurrent=0  Capacitance=1e-6  Setx0=off  InitialVoltage=0  Measurements=None
  Series RLC Branch5 : powerlib/Elements/Series RLC Branch  LConnTagsString=__new0  RConnTagsString=__new0  BranchType=L  Resistance=1  Inductance=1E-7  SetiL0=off  InitialCurrent=0  Capacitance=1e-6  Setx0=off  InitialVoltage=0  Measurements=None
  Series RLC Branch7 : powerlib/Elements/Series RLC Branch  LConnTagsString=__new0  RConnTagsString=__new0  BranchType=RL  Resistance=0.6  Inductance=1e-6  SetiL0=off  InitialCurrent=0  Capacitance=1e-6  Setx0=off  InitialVoltage=0  Measurements=None
  Series RLC Branch9 : powerlib/Elements/Series RLC Branch  LConnTagsString=__new0  RConnTagsString=__new0  BranchType=L  Resistance=1  Inductance=0.4e-6  SetiL0=off  InitialCurrent=0  Capacitance=1e-6  Setx0=off  InitialVoltage=0  Measurements=None
  Terminator{,1..9} (10 alike) : Terminator
  Udc+ : PMIOPort  Side=Left
  udc- : PMIOPort  Port=2  Side=Left
  p1 : PMIOPort  Port=3  Side=Right
  p2 : PMIOPort  Port=4  Side=Right
  wires:
  Demux/4 -> [n1]
  Demux/2 -> [p1]
  Demux/1 -> [p2]
  PWM/1 -> Demux/1
  Demux/3 -> [n2]
  Diode6/1 -> Terminator1/1
  Diode1/1 -> Terminator6/1
  Diode8/1 -> Terminator7/1
  [p2] -> IGBT/1
  Diode2/1 -> Terminator8/1
  Current Measurement1/1 -> Terminator/1
  [p1] -> IGBT2/1
  [n2] -> IGBT1/1
  IGBT/1 -> Terminator2/1
  IGBT2/1 -> Terminator3/1
  IGBT1/1 -> Terminator4/1
  [n1] -> IGBT3/1
  IGBT3/1 -> Terminator5/1
  Diode3/1 -> Terminator9/1
  connections:
  Diode1/RConn1 -- IGBT/RConn1 -- Diode8/LConn1 -- p2/RConn1 -- IGBT1/LConn1
  Series RLC Branch9/RConn1 -- Series RLC Branch7/LConn1 -- Series RLC Branch1/LConn1
  Series RLC Branch2/RConn1 -- Series RLC Branch10/RConn1 -- Series RLC Branch14/LConn1 -- Series RLC Branch5/LConn1
  Diode3/RConn1 -- IGBT2/RConn1 -- IGBT3/LConn1 -- p1/RConn1 -- Diode2/LConn1
  IGBT2/LConn1 -- Series RLC Branch12/RConn1 -- Diode2/RConn1
  Current Measurement1/RConn1 -- Diode6/LConn1
  Diode1/LConn1 -- Series RLC Branch5/RConn1 -- IGBT1/RConn1
  Diode8/RConn1 -- IGBT/LConn1 -- Series RLC Branch3/RConn1
  Diode3/LConn1 -- Series RLC Branch14/RConn1 -- IGBT3/RConn1
  Series RLC Branch12/LConn1 -- Series RLC Branch3/LConn1 -- Series RLC Branch1/RConn1 -- Current Measurement1/LConn1
  Series RLC Branch2/LConn1 -- Series RLC Branch7/RConn1 -- Diode6/RConn1
  Series RLC Branch9/LConn1 -- Udc+/RConn1
  Series RLC Branch10/LConn1 -- udc-/RConn1

== system model_sim_CHB5_36_new_temp/Subsystem/IGCT3 ==
  PWM : Inport
  Current Measurement1 : powerlib/Measurements/Current Measurement  PhasorSimulation=off  OutputType=Complex  PSBequivalent=0
  Demux : Demux
  Diode{1..3,6,8} (5 alike) : powerlib/Power Electronics/Diode  Ron=DIODE.rF  Lon=0  Vf=DIODE.VF0  IC=0  UseSnubber=off  Rs=500  Cs=250e-9  Measurements=on
  IGBT{,1..3} (4 alike) : powerlib/Power Electronics/IGBT  Ron=IGCT.rT  Lon=0  Vf=IGCT.VT0  Tf=1e-6  Tt=2e-6  IC=0  Rs=1e5  Cs=inf  Measurements=on
  Series RLC Branch1 : powerlib/Elements/Series RLC Branch  LConnTagsString=__new0  RConnTagsString=__new0  BranchType=RL  Resistance=1e-5  Inductance=3.0E-6  SetiL0=off  InitialCurrent=0  Capacitance=1e-6  Setx0=off  InitialVoltage=0  Measurements=None
  Series RLC Branch10 : powerlib/Elements/Series RLC Branch  LConnTagsString=__new0  RConnTagsString=__new0  BranchType=L  Resistance=1  Inductance=0.4e-6  SetiL0=off  InitialCurrent=0  Capacitance=1e-6  Setx0=off  InitialVoltage=0  Measurements=None
  Series RLC Branch12 : powerlib/Elements/Series RLC Branch  LConnTagsString=__new0  RConnTagsString=__new0  BranchType=RL  Resistance=1e-5  Inductance=1E-9  SetiL0=off  InitialCurrent=0  Capacitance=1e-6  Setx0=off  InitialVoltage=0  Measurements=None
  Series RLC Branch14 : powerlib/Elements/Series RLC Branch  LConnTagsString=__new0  RConnTagsString=__new0  BranchType=L  Resistance=1  Inductance=1E-7  SetiL0=off  InitialCurrent=0  Capacitance=1e-6  Setx0=off  InitialVoltage=0  Measurements=None
  Series RLC Branch2 : powerlib/Elements/Series RLC Branch  LConnTagsString=__new0  RConnTagsString=__new0  BranchType=RC  Resistance=1e-5  Inductance=20e-6  SetiL0=off  InitialCurrent=0  Capacitance=17e-6  Setx0=off  InitialVoltage=0  Measurements=None
  Series RLC Branch3 : powerlib/Elements/Series RLC Branch  LConnTagsString=__new0  RConnTagsString=__new0  BranchType=RL  Resistance=1e-5  Inductance=1E-9  SetiL0=off  InitialCurrent=0  Capacitance=1e-6  Setx0=off  InitialVoltage=0  Measurements=None
  Series RLC Branch5 : powerlib/Elements/Series RLC Branch  LConnTagsString=__new0  RConnTagsString=__new0  BranchType=L  Resistance=1  Inductance=1E-7  SetiL0=off  InitialCurrent=0  Capacitance=1e-6  Setx0=off  InitialVoltage=0  Measurements=None
  Series RLC Branch7 : powerlib/Elements/Series RLC Branch  LConnTagsString=__new0  RConnTagsString=__new0  BranchType=RL  Resistance=0.6  Inductance=1e-6  SetiL0=off  InitialCurrent=0  Capacitance=1e-6  Setx0=off  InitialVoltage=0  Measurements=None
  Series RLC Branch9 : powerlib/Elements/Series RLC Branch  LConnTagsString=__new0  RConnTagsString=__new0  BranchType=L  Resistance=1  Inductance=0.4e-6  SetiL0=off  InitialCurrent=0  Capacitance=1e-6  Setx0=off  InitialVoltage=0  Measurements=None
  Terminator{,1..9} (10 alike) : Terminator
  Udc+ : PMIOPort  Side=Left
  udc- : PMIOPort  Port=2  Side=Left
  p1 : PMIOPort  Port=3  Side=Right
  p2 : PMIOPort  Port=4  Side=Right
  wires:
  Diode3/1 -> Terminator9/1
  IGBT3/1 -> Terminator5/1
  [n1] -> IGBT3/1
  IGBT1/1 -> Terminator4/1
  IGBT2/1 -> Terminator3/1
  IGBT/1 -> Terminator2/1
  [n2] -> IGBT1/1
  [p1] -> IGBT2/1
  Current Measurement1/1 -> Terminator/1
  Diode2/1 -> Terminator8/1
  [p2] -> IGBT/1
  Diode8/1 -> Terminator7/1
  Diode1/1 -> Terminator6/1
  Diode6/1 -> Terminator1/1
  Demux/3 -> [n2]
  PWM/1 -> Demux/1
  Demux/1 -> [p2]
  Demux/2 -> [p1]
  Demux/4 -> [n1]
  connections:
  Series RLC Branch10/LConn1 -- udc-/RConn1
  Series RLC Branch9/LConn1 -- Udc+/RConn1
  Diode6/RConn1 -- Series RLC Branch7/RConn1 -- Series RLC Branch2/LConn1
  Current Measurement1/LConn1 -- Series RLC Branch1/RConn1 -- Series RLC Branch3/LConn1 -- Series RLC Branch12/LConn1
  IGBT3/RConn1 -- Series RLC Branch14/RConn1 -- Diode3/LConn1
  Series RLC Branch3/RConn1 -- IGBT/LConn1 -- Diode8/RConn1
  IGBT1/RConn1 -- Series RLC Branch5/RConn1 -- Diode1/LConn1
  Current Measurement1/RConn1 -- Diode6/LConn1
  Diode2/RConn1 -- Series RLC Branch12/RConn1 -- IGBT2/LConn1
  Diode2/LConn1 -- p1/RConn1 -- IGBT3/LConn1 -- IGBT2/RConn1 -- Diode3/RConn1
  Series RLC Branch5/LConn1 -- Series RLC Branch14/LConn1 -- Series RLC Branch10/RConn1 -- Series RLC Branch2/RConn1
  Series RLC Branch1/LConn1 -- Series RLC Branch7/LConn1 -- Series RLC Branch9/RConn1
  IGBT1/LConn1 -- p2/RConn1 -- Diode8/LConn1 -- IGBT/RConn1 -- Diode1/RConn1

== system model_sim_CHB5_36_new_temp/Subsystem/IGCT4 ==
  PWM : Inport
  Current Measurement1 : powerlib/Measurements/Current Measurement  PhasorSimulation=off  OutputType=Complex  PSBequivalent=0
  Demux : Demux
  Diode{1..3,6,8} (5 alike) : powerlib/Power Electronics/Diode  Ron=DIODE.rF  Lon=0  Vf=DIODE.VF0  IC=0  UseSnubber=off  Rs=500  Cs=250e-9  Measurements=on
  IGBT{,1..3} (4 alike) : powerlib/Power Electronics/IGBT  Ron=IGCT.rT  Lon=0  Vf=IGCT.VT0  Tf=1e-6  Tt=2e-6  IC=0  Rs=1e5  Cs=inf  Measurements=on
  Series RLC Branch1 : powerlib/Elements/Series RLC Branch  LConnTagsString=__new0  RConnTagsString=__new0  BranchType=RL  Resistance=1e-5  Inductance=3.0E-6  SetiL0=off  InitialCurrent=0  Capacitance=1e-6  Setx0=off  InitialVoltage=0  Measurements=None
  Series RLC Branch10 : powerlib/Elements/Series RLC Branch  LConnTagsString=__new0  RConnTagsString=__new0  BranchType=L  Resistance=1  Inductance=0.4e-6  SetiL0=off  InitialCurrent=0  Capacitance=1e-6  Setx0=off  InitialVoltage=0  Measurements=None
  Series RLC Branch12 : powerlib/Elements/Series RLC Branch  LConnTagsString=__new0  RConnTagsString=__new0  BranchType=RL  Resistance=1e-5  Inductance=1E-9  SetiL0=off  InitialCurrent=0  Capacitance=1e-6  Setx0=off  InitialVoltage=0  Measurements=None
  Series RLC Branch14 : powerlib/Elements/Series RLC Branch  LConnTagsString=__new0  RConnTagsString=__new0  BranchType=L  Resistance=1  Inductance=1E-7  SetiL0=off  InitialCurrent=0  Capacitance=1e-6  Setx0=off  InitialVoltage=0  Measurements=None
  Series RLC Branch2 : powerlib/Elements/Series RLC Branch  LConnTagsString=__new0  RConnTagsString=__new0  BranchType=RC  Resistance=1e-5  Inductance=20e-6  SetiL0=off  InitialCurrent=0  Capacitance=17e-6  Setx0=off  InitialVoltage=0  Measurements=None
  Series RLC Branch3 : powerlib/Elements/Series RLC Branch  LConnTagsString=__new0  RConnTagsString=__new0  BranchType=RL  Resistance=1e-5  Inductance=1E-9  SetiL0=off  InitialCurrent=0  Capacitance=1e-6  Setx0=off  InitialVoltage=0  Measurements=None
  Series RLC Branch5 : powerlib/Elements/Series RLC Branch  LConnTagsString=__new0  RConnTagsString=__new0  BranchType=L  Resistance=1  Inductance=1E-7  SetiL0=off  InitialCurrent=0  Capacitance=1e-6  Setx0=off  InitialVoltage=0  Measurements=None
  Series RLC Branch7 : powerlib/Elements/Series RLC Branch  LConnTagsString=__new0  RConnTagsString=__new0  BranchType=RL  Resistance=0.6  Inductance=1e-6  SetiL0=off  InitialCurrent=0  Capacitance=1e-6  Setx0=off  InitialVoltage=0  Measurements=None
  Series RLC Branch9 : powerlib/Elements/Series RLC Branch  LConnTagsString=__new0  RConnTagsString=__new0  BranchType=L  Resistance=1  Inductance=0.4e-6  SetiL0=off  InitialCurrent=0  Capacitance=1e-6  Setx0=off  InitialVoltage=0  Measurements=None
  Terminator{,1..9} (10 alike) : Terminator
  Udc+ : PMIOPort  Side=Left
  udc- : PMIOPort  Port=2  Side=Left
  p1 : PMIOPort  Port=3  Side=Right
  p2 : PMIOPort  Port=4  Side=Right
  wires:
  Demux/4 -> [n1]
  Demux/2 -> [p1]
  Demux/1 -> [p2]
  PWM/1 -> Demux/1
  Demux/3 -> [n2]
  Diode6/1 -> Terminator1/1
  Diode1/1 -> Terminator6/1
  Diode8/1 -> Terminator7/1
  [p2] -> IGBT/1
  Diode2/1 -> Terminator8/1
  Current Measurement1/1 -> Terminator/1
  [p1] -> IGBT2/1
  [n2] -> IGBT1/1
  IGBT/1 -> Terminator2/1
  IGBT2/1 -> Terminator3/1
  IGBT1/1 -> Terminator4/1
  [n1] -> IGBT3/1
  IGBT3/1 -> Terminator5/1
  Diode3/1 -> Terminator9/1
  connections:
  Diode1/RConn1 -- IGBT/RConn1 -- Diode8/LConn1 -- p2/RConn1 -- IGBT1/LConn1
  Series RLC Branch9/RConn1 -- Series RLC Branch7/LConn1 -- Series RLC Branch1/LConn1
  Series RLC Branch2/RConn1 -- Series RLC Branch10/RConn1 -- Series RLC Branch14/LConn1 -- Series RLC Branch5/LConn1
  Diode3/RConn1 -- IGBT2/RConn1 -- IGBT3/LConn1 -- p1/RConn1 -- Diode2/LConn1
  IGBT2/LConn1 -- Series RLC Branch12/RConn1 -- Diode2/RConn1
  Current Measurement1/RConn1 -- Diode6/LConn1
  Diode1/LConn1 -- Series RLC Branch5/RConn1 -- IGBT1/RConn1
  Diode8/RConn1 -- IGBT/LConn1 -- Series RLC Branch3/RConn1
  Diode3/LConn1 -- Series RLC Branch14/RConn1 -- IGBT3/RConn1
  Series RLC Branch12/LConn1 -- Series RLC Branch3/LConn1 -- Series RLC Branch1/RConn1 -- Current Measurement1/LConn1
  Series RLC Branch2/LConn1 -- Series RLC Branch7/RConn1 -- Diode6/RConn1
  Series RLC Branch9/LConn1 -- Udc+/RConn1
  Series RLC Branch10/LConn1 -- udc-/RConn1

== system model_sim_CHB5_36_new_temp/Subsystem/IGCT5 ==
  PWM : Inport
  Current Measurement1 : powerlib/Measurements/Current Measurement  PhasorSimulation=off  OutputType=Complex  PSBequivalent=0
  Demux : Demux
  Diode{1..3,6,8} (5 alike) : powerlib/Power Electronics/Diode  Ron=DIODE.rF  Lon=0  Vf=DIODE.VF0  IC=0  UseSnubber=off  Rs=500  Cs=250e-9  Measurements=on
  IGBT{,1..3} (4 alike) : powerlib/Power Electronics/IGBT  Ron=IGCT.rT  Lon=0  Vf=IGCT.VT0  Tf=1e-6  Tt=2e-6  IC=0  Rs=1e5  Cs=inf  Measurements=on
  Series RLC Branch1 : powerlib/Elements/Series RLC Branch  LConnTagsString=__new0  RConnTagsString=__new0  BranchType=RL  Resistance=1e-5  Inductance=3.0E-6  SetiL0=off  InitialCurrent=0  Capacitance=1e-6  Setx0=off  InitialVoltage=0  Measurements=None
  Series RLC Branch10 : powerlib/Elements/Series RLC Branch  LConnTagsString=__new0  RConnTagsString=__new0  BranchType=L  Resistance=1  Inductance=0.4e-6  SetiL0=off  InitialCurrent=0  Capacitance=1e-6  Setx0=off  InitialVoltage=0  Measurements=None
  Series RLC Branch12 : powerlib/Elements/Series RLC Branch  LConnTagsString=__new0  RConnTagsString=__new0  BranchType=RL  Resistance=1e-5  Inductance=1E-9  SetiL0=off  InitialCurrent=0  Capacitance=1e-6  Setx0=off  InitialVoltage=0  Measurements=None
  Series RLC Branch14 : powerlib/Elements/Series RLC Branch  LConnTagsString=__new0  RConnTagsString=__new0  BranchType=L  Resistance=1  Inductance=1E-7  SetiL0=off  InitialCurrent=0  Capacitance=1e-6  Setx0=off  InitialVoltage=0  Measurements=None
  Series RLC Branch2 : powerlib/Elements/Series RLC Branch  LConnTagsString=__new0  RConnTagsString=__new0  BranchType=RC  Resistance=1e-5  Inductance=20e-6  SetiL0=off  InitialCurrent=0  Capacitance=17e-6  Setx0=off  InitialVoltage=0  Measurements=None
  Series RLC Branch3 : powerlib/Elements/Series RLC Branch  LConnTagsString=__new0  RConnTagsString=__new0  BranchType=RL  Resistance=1e-5  Inductance=1E-9  SetiL0=off  InitialCurrent=0  Capacitance=1e-6  Setx0=off  InitialVoltage=0  Measurements=None
  Series RLC Branch5 : powerlib/Elements/Series RLC Branch  LConnTagsString=__new0  RConnTagsString=__new0  BranchType=L  Resistance=1  Inductance=1E-7  SetiL0=off  InitialCurrent=0  Capacitance=1e-6  Setx0=off  InitialVoltage=0  Measurements=None
  Series RLC Branch7 : powerlib/Elements/Series RLC Branch  LConnTagsString=__new0  RConnTagsString=__new0  BranchType=RL  Resistance=0.6  Inductance=1e-6  SetiL0=off  InitialCurrent=0  Capacitance=1e-6  Setx0=off  InitialVoltage=0  Measurements=None
  Series RLC Branch9 : powerlib/Elements/Series RLC Branch  LConnTagsString=__new0  RConnTagsString=__new0  BranchType=L  Resistance=1  Inductance=0.4e-6  SetiL0=off  InitialCurrent=0  Capacitance=1e-6  Setx0=off  InitialVoltage=0  Measurements=None
  Terminator{,1..9} (10 alike) : Terminator
  Udc+ : PMIOPort  Side=Left
  udc- : PMIOPort  Port=2  Side=Left
  p1 : PMIOPort  Port=3  Side=Right
  p2 : PMIOPort  Port=4  Side=Right
  wires:
  Diode3/1 -> Terminator9/1
  IGBT3/1 -> Terminator5/1
  [n1] -> IGBT3/1
  IGBT1/1 -> Terminator4/1
  IGBT2/1 -> Terminator3/1
  IGBT/1 -> Terminator2/1
  [n2] -> IGBT1/1
  [p1] -> IGBT2/1
  Current Measurement1/1 -> Terminator/1
  Diode2/1 -> Terminator8/1
  [p2] -> IGBT/1
  Diode8/1 -> Terminator7/1
  Diode1/1 -> Terminator6/1
  Diode6/1 -> Terminator1/1
  Demux/3 -> [n2]
  PWM/1 -> Demux/1
  Demux/1 -> [p2]
  Demux/2 -> [p1]
  Demux/4 -> [n1]
  connections:
  Series RLC Branch10/LConn1 -- udc-/RConn1
  Series RLC Branch9/LConn1 -- Udc+/RConn1
  Diode6/RConn1 -- Series RLC Branch7/RConn1 -- Series RLC Branch2/LConn1
  Current Measurement1/LConn1 -- Series RLC Branch1/RConn1 -- Series RLC Branch3/LConn1 -- Series RLC Branch12/LConn1
  IGBT3/RConn1 -- Series RLC Branch14/RConn1 -- Diode3/LConn1
  Series RLC Branch3/RConn1 -- IGBT/LConn1 -- Diode8/RConn1
  IGBT1/RConn1 -- Series RLC Branch5/RConn1 -- Diode1/LConn1
  Current Measurement1/RConn1 -- Diode6/LConn1
  Diode2/RConn1 -- Series RLC Branch12/RConn1 -- IGBT2/LConn1
  Diode2/LConn1 -- p1/RConn1 -- IGBT3/LConn1 -- IGBT2/RConn1 -- Diode3/RConn1
  Series RLC Branch5/LConn1 -- Series RLC Branch14/LConn1 -- Series RLC Branch10/RConn1 -- Series RLC Branch2/RConn1
  Series RLC Branch1/LConn1 -- Series RLC Branch7/LConn1 -- Series RLC Branch9/RConn1
  IGBT1/LConn1 -- p2/RConn1 -- Diode8/LConn1 -- IGBT/RConn1 -- Diode1/RConn1

== system model_sim_CHB5_36_new_temp/Subsystem/IGCT6 ==
  PWM : Inport
  Current Measurement1 : powerlib/Measurements/Current Measurement  PhasorSimulation=off  OutputType=Complex  PSBequivalent=0
  Demux : Demux
  Diode{1..3,6,8} (5 alike) : powerlib/Power Electronics/Diode  Ron=DIODE.rF  Lon=0  Vf=DIODE.VF0  IC=0  UseSnubber=off  Rs=500  Cs=250e-9  Measurements=on
  IGBT{,1..3} (4 alike) : powerlib/Power Electronics/IGBT  Ron=IGCT.rT  Lon=0  Vf=IGCT.VT0  Tf=1e-6  Tt=2e-6  IC=0  Rs=1e5  Cs=inf  Measurements=on
  Series RLC Branch1 : powerlib/Elements/Series RLC Branch  LConnTagsString=__new0  RConnTagsString=__new0  BranchType=RL  Resistance=1e-5  Inductance=3.0E-6  SetiL0=off  InitialCurrent=0  Capacitance=1e-6  Setx0=off  InitialVoltage=0  Measurements=None
  Series RLC Branch10 : powerlib/Elements/Series RLC Branch  LConnTagsString=__new0  RConnTagsString=__new0  BranchType=L  Resistance=1  Inductance=0.4e-6  SetiL0=off  InitialCurrent=0  Capacitance=1e-6  Setx0=off  InitialVoltage=0  Measurements=None
  Series RLC Branch12 : powerlib/Elements/Series RLC Branch  LConnTagsString=__new0  RConnTagsString=__new0  BranchType=RL  Resistance=1e-5  Inductance=1E-9  SetiL0=off  InitialCurrent=0  Capacitance=1e-6  Setx0=off  InitialVoltage=0  Measurements=None
  Series RLC Branch14 : powerlib/Elements/Series RLC Branch  LConnTagsString=__new0  RConnTagsString=__new0  BranchType=L  Resistance=1  Inductance=1E-7  SetiL0=off  InitialCurrent=0  Capacitance=1e-6  Setx0=off  InitialVoltage=0  Measurements=None
  Series RLC Branch2 : powerlib/Elements/Series RLC Branch  LConnTagsString=__new0  RConnTagsString=__new0  BranchType=RC  Resistance=1e-5  Inductance=20e-6  SetiL0=off  InitialCurrent=0  Capacitance=17e-6  Setx0=off  InitialVoltage=0  Measurements=None
  Series RLC Branch3 : powerlib/Elements/Series RLC Branch  LConnTagsString=__new0  RConnTagsString=__new0  BranchType=RL  Resistance=1e-5  Inductance=1E-9  SetiL0=off  InitialCurrent=0  Capacitance=1e-6  Setx0=off  InitialVoltage=0  Measurements=None
  Series RLC Branch5 : powerlib/Elements/Series RLC Branch  LConnTagsString=__new0  RConnTagsString=__new0  BranchType=L  Resistance=1  Inductance=1E-7  SetiL0=off  InitialCurrent=0  Capacitance=1e-6  Setx0=off  InitialVoltage=0  Measurements=None
  Series RLC Branch7 : powerlib/Elements/Series RLC Branch  LConnTagsString=__new0  RConnTagsString=__new0  BranchType=RL  Resistance=0.6  Inductance=1e-6  SetiL0=off  InitialCurrent=0  Capacitance=1e-6  Setx0=off  InitialVoltage=0  Measurements=None
  Series RLC Branch9 : powerlib/Elements/Series RLC Branch  LConnTagsString=__new0  RConnTagsString=__new0  BranchType=L  Resistance=1  Inductance=0.4e-6  SetiL0=off  InitialCurrent=0  Capacitance=1e-6  Setx0=off  InitialVoltage=0  Measurements=None
  Terminator{,1..9} (10 alike) : Terminator
  Udc+ : PMIOPort  Side=Left
  udc- : PMIOPort  Port=2  Side=Left
  p1 : PMIOPort  Port=3  Side=Right
  p2 : PMIOPort  Port=4  Side=Right
  wires:
  Demux/4 -> [n1]
  Demux/2 -> [p1]
  Demux/1 -> [p2]
  PWM/1 -> Demux/1
  Demux/3 -> [n2]
  Diode6/1 -> Terminator1/1
  Diode1/1 -> Terminator6/1
  Diode8/1 -> Terminator7/1
  [p2] -> IGBT/1
  Diode2/1 -> Terminator8/1
  Current Measurement1/1 -> Terminator/1
  [p1] -> IGBT2/1
  [n2] -> IGBT1/1
  IGBT/1 -> Terminator2/1
  IGBT2/1 -> Terminator3/1
  IGBT1/1 -> Terminator4/1
  [n1] -> IGBT3/1
  IGBT3/1 -> Terminator5/1
  Diode3/1 -> Terminator9/1
  connections:
  Diode1/RConn1 -- IGBT/RConn1 -- Diode8/LConn1 -- p2/RConn1 -- IGBT1/LConn1
  Series RLC Branch9/RConn1 -- Series RLC Branch7/LConn1 -- Series RLC Branch1/LConn1
  Series RLC Branch2/RConn1 -- Series RLC Branch10/RConn1 -- Series RLC Branch14/LConn1 -- Series RLC Branch5/LConn1
  Diode3/RConn1 -- IGBT2/RConn1 -- IGBT3/LConn1 -- p1/RConn1 -- Diode2/LConn1
  IGBT2/LConn1 -- Series RLC Branch12/RConn1 -- Diode2/RConn1
  Current Measurement1/RConn1 -- Diode6/LConn1
  Diode1/LConn1 -- Series RLC Branch5/RConn1 -- IGBT1/RConn1
  Diode8/RConn1 -- IGBT/LConn1 -- Series RLC Branch3/RConn1
  Diode3/LConn1 -- Series RLC Branch14/RConn1 -- IGBT3/RConn1
  Series RLC Branch12/LConn1 -- Series RLC Branch3/LConn1 -- Series RLC Branch1/RConn1 -- Current Measurement1/LConn1
  Series RLC Branch2/LConn1 -- Series RLC Branch7/RConn1 -- Diode6/RConn1
  Series RLC Branch9/LConn1 -- Udc+/RConn1
  Series RLC Branch10/LConn1 -- udc-/RConn1

== system model_sim_CHB5_36_new_temp/Subsystem3/DIODE ==
  I : Inport
  PWM1 : Inport  Port=2
  PWM2 : Inport  Port=3
  PWM3 : Inport  Port=4
  PWM4 : Inport  Port=5
  DIODE_204520 : Subsystem  VariantControl=DIODE_TP ==1  mask{DIODE=DIODE_204520}
      mask DialogControl ParameterGroupVar Prompt: DEVICE
  DIODE_344520 : Subsystem  VariantControl=DIODE_TP ==2  mask{DIODE=DIODE_344520}
      mask DialogControl ParameterGroupVar Prompt: DEVICE
  DIODE_D1031SH : Subsystem  VariantControl=DIODE_TP ==3  mask{DIODE=DIODE_D1031SH}
      mask DialogControl ParameterGroupVar Prompt: DEVICE
  DIODE_D1331SH : Subsystem  VariantControl=DIODE_TP ==4  mask{DIODE=DIODE_D1331SH}
      mask DialogControl ParameterGroupVar Prompt: DEVICE
  D1_BUS : Outport
  D2_BUS : Outport  Port=2
  D1_LOSS_MEAN : Outport  Port=3
  D2_LOSS_MEAN : Outport  Port=4
  D1_TEMP : Outport  Port=5
  D2_TEMP : Outport  Port=6
  TEMLIM_BOOL : Outport  Port=7

== system model_sim_CHB5_36_new_temp/Subsystem3/IGCT ==
  I : Inport
  PWM1 : Inport  Port=2
  PWM2 : Inport  Port=3
  IGCT_364520_36 : Subsystem  VariantControl=IGCTTP == 1  mask{IGCT=IGCT_364520_36}
      mask DialogControl ParameterGroupVar Prompt: DEVICE
  IGCT_364521_36 : Subsystem  VariantControl=IGCTTP == 2  mask{IGCT=IGCT_364521_36}
      mask DialogControl ParameterGroupVar Prompt: DEVICE
  IGCT_654522_6 : Subsystem  VariantControl=IGCTTP == 3  mask{IGCT=IGCT_654522_6}
      mask DialogControl ParameterGroupVar Prompt: DEVICE
  T1_BUS : Outport
  T2_BUS : Outport  Port=2
  <T1_TEMP> : Outport  Port=3
  <T2_TEMP> : Outport  Port=4
  <T1_LOSS_MEAN> : Outport  Port=5
  <T2_LOSS_MEAN> : Outport  Port=6
  TEMLIM_BOOL : Outport  Port=7
